simulink model "v1_VoltageImitator_PID"  (R2020b)
settings: Solver=ode23t  StartTime=0.0  StopTime=0.25  RelTol=1e-3
libraries: powerlib x10, pid_lib x1, simulink x1
settings Model: Creator=Александр  LastModifiedBy=Александр

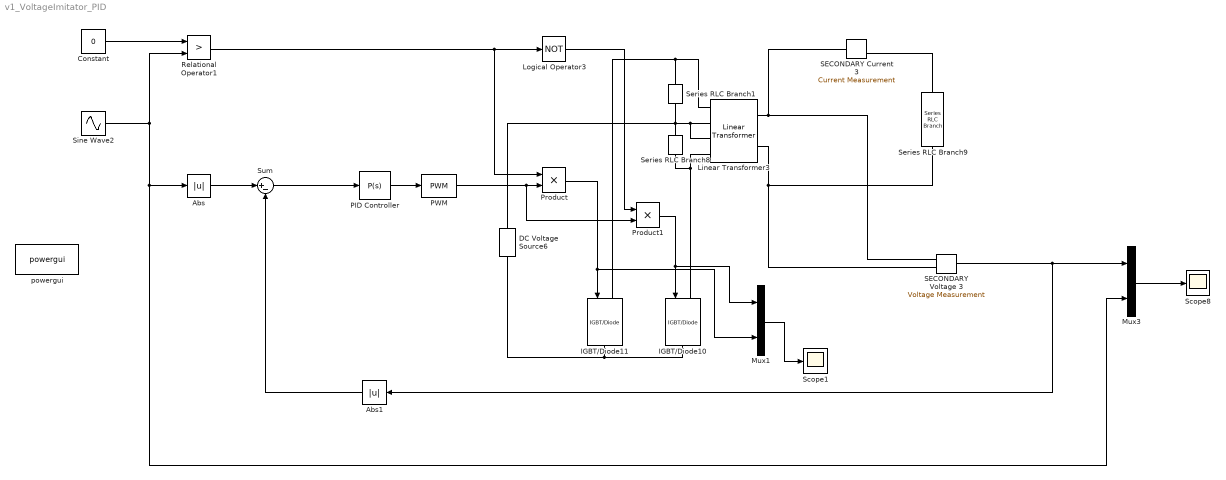
== system v1_VoltageImitator_PID ==
  Abs : Abs
  Abs1 : Abs
  Constant : Constant  Value=0
  DC Voltage Source6 : powerlib/Electrical Sources/DC Voltage Source  Amplitude=12  Measurements=None
  IGBT/Diode10 : powerlib/Power Electronics/IGBT//Diode  Ron=1e-3  Rs=1e5  Cs=inf  Measurements=off
  IGBT/Diode11 : powerlib/Power Electronics/IGBT//Diode  Ron=1e-3  Rs=1e5  Cs=inf  Measurements=off
  Linear Transformer3 : powerlib/Elements/Linear Transformer  UNITS=SI  NominalPower=[1.5 50 ]  winding1=[220 2950 2.2]  winding2=[12 43.2 10.4e-3]  ThreeWindings=on  winding3=[12 43.2 10.4e-3]  RmLm=[50e3 500]  Measurements=None  DataType=on
  Logical Operator3 : Logic  Operator=NOT  IconShape=distinctive  AllPortsSameDT=off  OutDataTypeStr=boolean
  Mux1 : Mux  Inputs=2
  Mux3 : Mux  Inputs=2
  PID Controller : pid_lib/PID Controller  Controller=P  Form=Parallel  TimeDomain=Continuous-time  UseExternalTs=off  SampleTime=-1  IntegratorMethod=Forward Euler  FilterMethod=Forward Euler  ControllerParametersSource=internal  P=0.5  I=0  D=0.00001  UseFilter=on  N=19208  TunerSelectOption=Transfer Function Based (PID Tuner App)  ZeroCross=off  InitialConditionSource=internal  InitialConditionForIntegrator=0  InitialConditionForFilter=0  DifferentiatorICPrevScaledInput=0  ExternalReset=none  TrackingMode=off  Kt=1  LimitOutput=off  SatLimitsSource=internal  UpperSaturationLimit=0.95  LowerSaturationLimit=0.5  LinearizeAsGain=on  AntiWindupMode=none  Kb=1  POutMin=[]  POutMax=[]  IOutMin=[]  IOutMax=[]  DOutMin=[]  DOutMax=[]  NOutMin=[]  NOutMax=[]  SumOutMin=[]  SumOutMax=[]  SaturationOutMin=[]  SaturationOutMax=[]  PParamMin=[]  PParamMax=[]  IParamMin=[]  IParamMax=[]  DParamMin=[]  DParamMax=[]  NParamMin=[]  NParamMax=[]  KbParamMin=[]  KbParamMax=[]  KtParamMin=[]  KtParamMax=[]  KbOutMin=[]  KbOutMax=[]  KtOutMin=[]  KtOutMax=[]  IntegratorOutMin=[]  IntegratorOutMax=[]  FilterOutMin=[]  FilterOutMax=[]  SumI1OutMin=[]  SumI1OutMax=[]  SumI2OutMin=[]  SumI2OutMax=[]  SumI3OutMin=[]  SumI3OutMax=[]  SumI4OutMin=[]  SumI4OutMax=[]  SumDOutMin=[]  SumDOutMax=[]  DifferentiatorOutMin=[]  DifferentiatorOutMax=[]  FilterDiffOutCoefMin=[]  FilterDiffOutCoefMax=[]  ReciprocalOutMin=[]  ReciprocalOutMax=[]  SumDenOutMin=[]  SumDenOutMax=[]  SumNumOutMin=[]  SumNumOutMax=[]  DivideOutMin=[]  DivideOutMax=[]  UdiffTsProdOutMin=[]  UdiffTsProdOutMax=[]  NTsProdOutMin=[]  NTsProdOutMax=[]  UintegralTsProdOutMin=[]  UintegralTsProdOutMax=[]  UngainTsProdOutMin=[]  UngainTsProdOutMax=[]  IntegratorContinuousStateAttributes=''  IntegratorStateMustResolveToSignalObject=off  IntegratorRTWStateStorageClass=Auto  FilterContinuousStateAttributes=''  FilterStateMustResolveToSignalObject=off  FilterRTWStateStorageClass=Auto  ParallelPVariant=InternalParameters  IdealPVariant=Disabled  IVariant=Disabled  DVariant=Disabled  IntegratorVariant=Disabled  SatVariant=Disabled  AWVariant=Disabled  PCopyVariant=Disabled  TRVariant=Disabled  FdbkBlocksVariant=Forward  IdealPFdbkVariant=Disabled  SatFdbkVariant=Disabled  DerivativeFilterVariant=Disabled  NVariant=Disabled  NCopyVariant=Disabled_SignalSpec  FilterICVariant=Disabled  IntegratorICVariant=Disabled  ExternalResetVariant=Disabled  TRSumVariant=Passthrough  SumFdbkVariant=Disabled  SumVariant=Passthrough_P  TsampFilterVariant=InternalTs  TsampNgainVariant=Passthrough  TsampIntegralVariant=Disabled_SignalSpec  ExternalSaturationOutDataTypeStr=Inherit: Same as second input
  PWM : simulink/Discontinuities/PWM  DisableCoverage=on  Period=1/100e3  DisallowZeroDutyCycle=off  RunAtFixedTimeIntervals=off  SampleTime=0.1
  Product : Product
  Product1 : Product
  Relational Operator1 : RelationalOperator  Operator=>  OutDataTypeStr=boolean  RndMeth=Nearest
  SECONDARY Current 3 : powerlib/Measurements/Current Measurement  PhasorSimulation=off  OutputType=Complex  PSBequivalent=0
  SECONDARY Voltage 3 : powerlib/Measurements/Voltage Measurement  PhasorSimulation=off  OutputType=Complex  PSBequivalent=0
  Scope1 : Scope
  Scope8 : Scope
  Series RLC Branch1 : powerlib/Elements/Series RLC Branch  LConnTagsString=__new0  RConnTagsString=__new0  BranchType=RC  Resistance=10  Inductance=50e-3  SetiL0=off  InitialCurrent=0  Capacitance=10e-6  Setx0=off  InitialVoltage=0  Measurements=None
  Series RLC Branch8 : powerlib/Elements/Series RLC Branch  LConnTagsString=__new0  RConnTagsString=__new0  BranchType=RC  Resistance=10  Inductance=50e-3  SetiL0=off  InitialCurrent=0  Capacitance=10e-6  Setx0=off  InitialVoltage=0  Measurements=None
  Series RLC Branch9 : powerlib/Elements/Series RLC Branch  LConnTagsString=__new0  RConnTagsString=__new0  BranchType=R  Resistance=100000  Inductance=1e-3  SetiL0=off  InitialCurrent=0  Capacitance=1e-6  Setx0=off  InitialVoltage=0  Measurements=None
  Sine Wave2 : Sin  Amplitude=100  Frequency=2*pi*50  SampleTime=0
  Sum : Sum  Inputs=|+-
  powergui : powerlib/powergui  Priority=1  SimulationMode=Continuous  SampleTime=50e-6  frequency=60  Iterations=50  frequencyindice=0  Pbase=100e6  ErrMax=1e-4  UnitsV=kV  UnitsW=MW  buscounter=0  FunctionMessages=off  echomessages=off  EnableUseOfTLC=off  CurrentSourceSwitches=off  DisableSnubberDevices=off  DisableRonSwitches=off  DisableVfSwitches=off  DisplayEquations=off  AutomaticDiscreteSolvers=off  SolverType=Tustin/Backward Euler (TBE)  Interpol=off  ExternalGateDelay=off  methode=off  Ts=100  x0status=blocks  SPID=on  SwTol=0  HookPort=off  NonlinearTolerance=1e-4  nMaxIteration=100  ContinueOnMaxIteration=off  RestoreLinks=warning  ResistiveCurrentMeasurement=off  Frange=[0:2:500]  Ylog=off  Xlog=on  ShowGrid=off  save=off  variable=ZData  structure=0  ZoomFFT=off  StartTime=0.0  cycles=1  DisplayStyle=1  fundamental=60  FreqAxis=off  MaxFrequency=1000  frequencyindicesteady=1  RmsSteady=1  display=off
  wires:
  Mux3/1 -> Scope8/1
  Constant/1 -> Relational Operator1/1
  Sine Wave2/1 -> Relational Operator1/2, Mux3/2, Abs/1
  PWM/1 -> Product1/2, Product/2
  Relational Operator1/1 -> Product/1, Logical Operator3/1
  Product/1 -> Mux1/2, IGBT/Diode11/1
  Product1/1 -> Mux1/1, IGBT/Diode10/1
  Logical Operator3/1 -> Product1/1
  SECONDARY Voltage 3/1 -> Mux3/1, Abs1/1
  Mux1/1 -> Scope1/1
  PID Controller/1 -> PWM/1
  Sum/1 -> PID Controller/1
  Abs/1 -> Sum/1
  Abs1/1 -> Sum/2
  connections:
  Linear Transformer3/LConn2 -- SECONDARY Voltage 3/LConn2 -- Series RLC Branch9/RConn1
  Linear Transformer3/RConn2 -- Series RLC Branch1/RConn1 -- Series RLC Branch8/LConn1 -- DC Voltage Source6/RConn1 -- Linear Transformer3/RConn3
  IGBT/Diode10/LConn1 -- Series RLC Branch8/RConn1 -- Linear Transformer3/RConn4
  Linear Transformer3/LConn1 -- SECONDARY Voltage 3/LConn1 -- SECONDARY Current 3/LConn1
  IGBT/Diode11/LConn1 -- Series RLC Branch1/LConn1 -- Linear Transformer3/RConn1
  SECONDARY Current 3/RConn1 -- Series RLC Branch9/LConn1
  IGBT/Diode10/RConn1 -- DC Voltage Source6/LConn1 -- IGBT/Diode11/RConn1
